simulink model "step_2"  (R2020a)
settings: Solver=VariableStepAuto  StartTime=0.0  StopTime=5  RelTol=1e-3
libraries: simulink x1
settings Model: Creator=HP  LastModifiedBy=HP

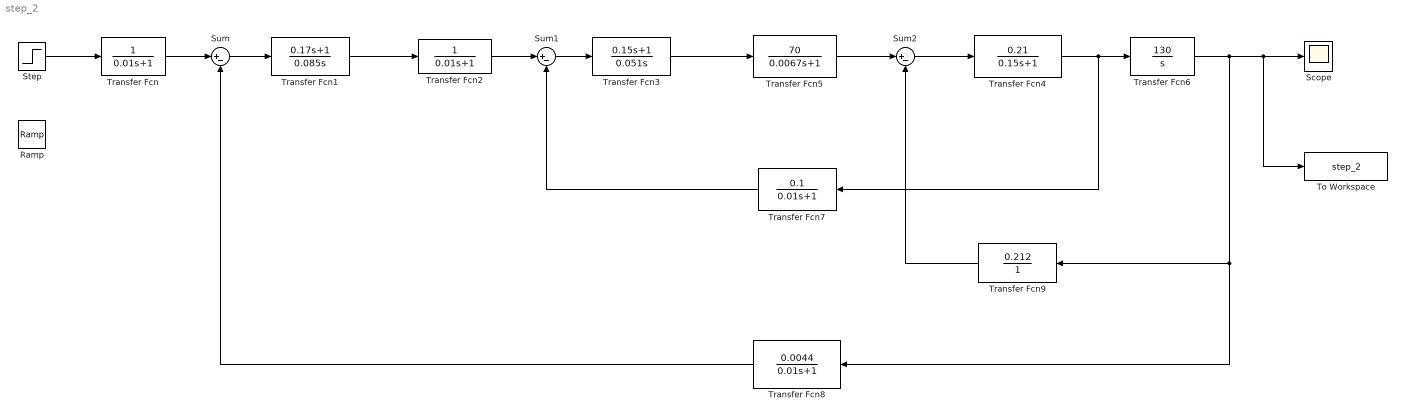
== system step_2 ==
  Ramp : simulink/Sources/Ramp  slope=1  start=0  InitialOutput=0
  Scope : Scope
  Step : Step  Time=0  SampleTime=0
  Sum : Sum  Inputs=|+-
  Sum1 : Sum  Inputs=|+-
  Sum2 : Sum  Inputs=|+-
  To Workspace : ToWorkspace  VariableName=step_2  SampleTime=0.001
  Transfer Fcn : TransferFcn  Denominator=[0.01 1]
  Transfer Fcn1 : TransferFcn  Numerator=[0.17 1]  Denominator=[0.085 0]
  Transfer Fcn2 : TransferFcn  Denominator=[0.01 1]
  Transfer Fcn3 : TransferFcn  Numerator=[0.15 1]  Denominator=[0.051 0]
  Transfer Fcn4 : TransferFcn  Numerator=[0.21]  Denominator=[0.15 1]
  Transfer Fcn5 : TransferFcn  Numerator=[70]  Denominator=[0.0067 1]
  Transfer Fcn6 : TransferFcn  Numerator=[130]  Denominator=[1 0]
  Transfer Fcn7 : TransferFcn  Numerator=[0.1]  Denominator=[0.01 1]
  Transfer Fcn8 : TransferFcn  Numerator=[0.0044]  Denominator=[0.01 1]
  Transfer Fcn9 : TransferFcn  Numerator=[0.212]  Denominator=[1]
  wires:
  Sum/1 -> Transfer Fcn1/1
  Transfer Fcn/1 -> Sum/1
  Transfer Fcn1/1 -> Transfer Fcn2/1
  Transfer Fcn3/1 -> Transfer Fcn5/1
  Sum1/1 -> Transfer Fcn3/1
  Transfer Fcn2/1 -> Sum1/1
  Sum2/1 -> Transfer Fcn4/1
  Transfer Fcn5/1 -> Sum2/1
  Transfer Fcn4/1 -> Transfer Fcn7/1, Transfer Fcn6/1
  Transfer Fcn7/1 -> Sum1/2
  Step/1 -> Transfer Fcn/1
  Transfer Fcn6/1 -> Transfer Fcn8/1, Transfer Fcn9/1, To Workspace/1, Scope/1
  Transfer Fcn9/1 -> Sum2/2
  Transfer Fcn8/1 -> Sum/2
